simulink model "Automatic_Power_Factor_Correction"  (R2021a)
settings: Solver=ode23tb  StartTime=0.0  StopTime=0.2  RelTol=1e-3
undefined symbols (not defined in the file): D1, Delta
libraries: spsThreePhaseParallelRLCLoadLib x4, spsThreePhaseBreakerLib x3, spsThreePhaseTransformerTwoWindingsLib x1, spsThreePhaseSourceLib x1, spsPower3phInstantaneousLib x1, spsThreePhaseVIMeasurementLib x1, spspowerguiLib x1
settings Model: Creator=thosiba  LastModifiedBy=saman
settings SolverCC: AlgebraicLoopSolver=TrustRegion
settings DataIOCC: ReturnWorkspaceOutputs=off
settings OptimizationCC: LifeSpan=inf
settings DebuggingCC: SFMachineParentedDataDiag=warning  ArithmeticOperatorsInVariantConditions=warning
settings HardwareCC: ProdBitPerSizeT=32  ProdBitPerPtrDiffT=32  ProdWordSize=32  ProdHWDeviceType=Specified
settings SFSimCC: SimUseLocalCustomCode=off  CustomCodeUndefinedFunction=UseInterfaceOnly
settings RTWCC: RTWUseLocalCustomCode=off
settings CodeAppCC: StateflowObjectComments=on
settings SimscapeCC: SimscapeNormalizeSystem=off

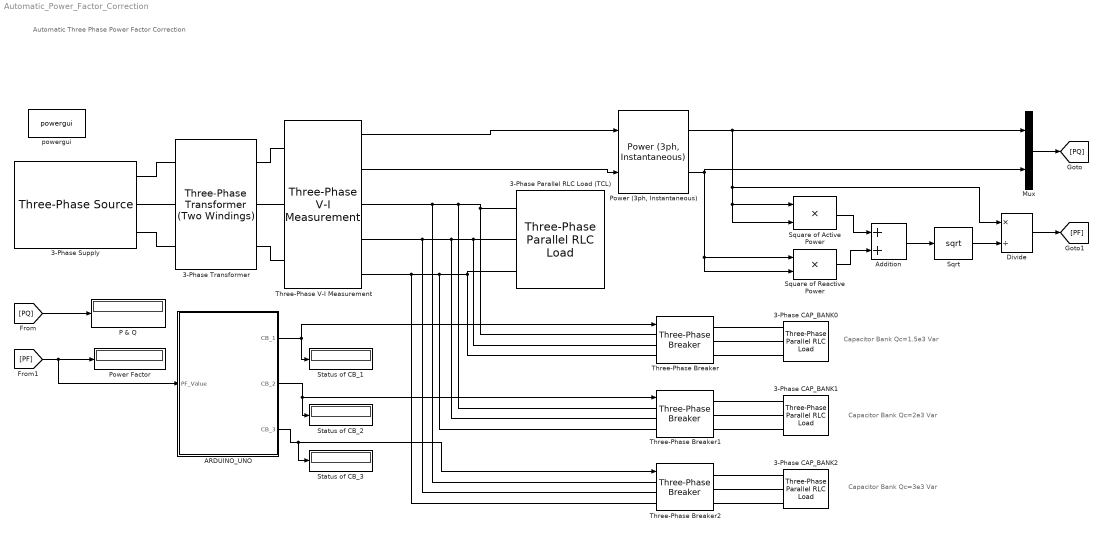
== system Automatic_Power_Factor_Correction ==
  note: Automatic Three Phase Power Factor Correction
  note: Capacitor Bank Qc=1.5e3 Var
  note: Capacitor Bank Qc=2e3 Var
  note: Capacitor Bank Qc=3e3 Var
  3-Phase CAP_BANK0 : spsThreePhaseParallelRLCLoadLib/Three-Phase Parallel RLC Load  LConnTagsString=A|B|C  Configuration=Y (grounded)  NominalVoltage=400  Vabc=[1e3 1e3 1e3]  Vabcp=[1e3 1e3 1e3]  NominalFrequency=50  UnbalancedPower=off  ActivePower=0  InductivePower=0  CapacitivePower=1.5e3  Pabc=[10e3 9e3 11e3]  QLabc=[100 90 110]  QCabc=[100 90 110]  Pabcp=[10e3 9e3 11e3]  QLabcp=[100 90 110]  QCabcp=[100 90 110]  Measurements=None  LoadType=constant PQ
  3-Phase CAP_BANK1 : spsThreePhaseParallelRLCLoadLib/Three-Phase Parallel RLC Load  LConnTagsString=A|B|C  Configuration=Y (grounded)  NominalVoltage=400  Vabc=[1e3 1e3 1e3]  Vabcp=[1e3 1e3 1e3]  NominalFrequency=50  UnbalancedPower=off  ActivePower=0  InductivePower=0  CapacitivePower=2e3  Pabc=[10e3 9e3 11e3]  QLabc=[100 90 110]  QCabc=[100 90 110]  Pabcp=[10e3 9e3 11e3]  QLabcp=[100 90 110]  QCabcp=[100 90 110]  Measurements=None  LoadType=constant PQ
  3-Phase CAP_BANK2 : spsThreePhaseParallelRLCLoadLib/Three-Phase Parallel RLC Load  LConnTagsString=A|B|C  Configuration=Y (grounded)  NominalVoltage=400  Vabc=[1e3 1e3 1e3]  Vabcp=[1e3 1e3 1e3]  NominalFrequency=50  UnbalancedPower=off  ActivePower=0  InductivePower=0  CapacitivePower=3e3  Pabc=[10e3 9e3 11e3]  QLabc=[100 90 110]  QCabc=[100 90 110]  Pabcp=[10e3 9e3 11e3]  QLabcp=[100 90 110]  QCabcp=[100 90 110]  Measurements=None  LoadType=constant PQ
  3-Phase Parallel RLC Load (TCL) : spsThreePhaseParallelRLCLoadLib/Three-Phase Parallel RLC Load  LConnTagsString=A|B|C  Configuration=Y (grounded)  NominalVoltage=400  Vabc=[1e3 1e3 1e3]  Vabcp=[1e3 1e3 1e3]  NominalFrequency=50  UnbalancedPower=off  ActivePower=5e3  InductivePower=7e3  CapacitivePower=0  Pabc=[10e3 9e3 11e3]  QLabc=[100 90 110]  QCabc=[100 90 110]  Pabcp=[10e3 9e3 11e3]  QLabcp=[100 90 110]  QCabcp=[100 90 110]  Measurements=None  LoadType=constant PQ
  "3-Phase Transformer " : spsThreePhaseTransformerTwoWindingsLib/Three-Phase Transformer (Two Windings)  Winding1Connection=Delta (D1)  Winding2Connection=Yg  CoreType=Three single-phase transformers  SetSaturation=off  Hysteresis=off  DataFile='hysteresis'  SetInitialFlux=off  Measurements=None  UNITS=pu  NominalPower=[ 1e6 , 50 ]  Winding1=[ 11e3 , 0.002 , 0.08 ]  Winding2=[ 400 , 0.002 , 0.08 ]  Rm=500  Lm=500  L0=0.5  Saturation=[ 0,0 ; 0.0024,1.2 ; 1.0,1.52 ]  InitialFluxes=[ 0.8 , -0.8 , 0.7 ]  BreakLoop=off  DiscreteSolver=Trapezoidal iterative  DataType=off  TransfoNumber=1
  3-Phase Supply : spsThreePhaseSourceLib/Three-Phase Source  InternalConnection=Yg  VoltagePhases=off  Voltage=11e3  PhaseAngle=0  Voltage_phases=[25e3 25e3 25e3]/sqrt(3)  PhaseAngles_phases=[0 -120 +120]  Frequency=50  NonIdealSource=on  SpecifyImpedance=on  Resistance=0.8929  Inductance=16.58e-3  ShortCircuitLevel=30e6  BaseVoltage=11e3  XRratio=7  BusType=swing  Pref=10e3  Qref=0  Prefabc=[10e3, 10e3, 10e3]  Qrefabc=[0, 0, 0]  Qmin=-inf  Qmax=inf
  ARDUINO_UNO : MATLAB Function  TreatAsAtomicUnit=on
  Addition : Sum
  Divide : Product  Inputs=*/
  Mux : Mux  Inputs=2
  P & Q : Display
      settings: Decimation=4
  "Power (3ph, Instantaneous)" : spsPower3phInstantaneousLib/Power (3ph, Instantaneous)
  Power Factor : Display
      settings: Decimation=4
  Sqrt : Sqrt  SaturateOnIntegerOverflow=on
  Square of Active Power : Product
  Square of Reactive Power : Product
  Status of CB_1 : Display
  Status of CB_2 : Display
  Status of CB_3 : Display
  Three-Phase V-I Measurement : spsThreePhaseVIMeasurementLib/Three-Phase V-I Measurement  VoltageMeasurement=phase-to-ground  SetLabelV=off  LabelV=Vabc  Vpu=off  VpuLL=off  CurrentMeasurement=yes  SetLabelI=off  LabelI=Iabc  Ipu=off  Pbase=100e6  Vbase=500e3  OutputType=Complex  PhasorSimulation=off  PSBequivalent=0
  Three-Phase Breaker : spsThreePhaseBreakerLib/Three-Phase Breaker  InitialState=open  SwitchA=on  SwitchB=on  SwitchC=on  SwitchTimes="[1/60  5/60]"  External=on  BreakerResistance=0.01  SnubberResistance=1e6  SnubberCapacitance=inf  Measurements=None
  Three-Phase Breaker1 : spsThreePhaseBreakerLib/Three-Phase Breaker  InitialState=open  SwitchA=on  SwitchB=on  SwitchC=on  SwitchTimes="[1/60  5/60]"  External=on  BreakerResistance=0.01  SnubberResistance=1e6  SnubberCapacitance=inf  Measurements=None
  Three-Phase Breaker2 : spsThreePhaseBreakerLib/Three-Phase Breaker  InitialState=open  SwitchA=on  SwitchB=on  SwitchC=on  SwitchTimes="[1/60  5/60]"  External=on  BreakerResistance=0.01  SnubberResistance=1e6  SnubberCapacitance=inf  Measurements=None
  powergui : spspowerguiLib/powergui  Priority=1  SimulationMode=Continuous  SampleTime=50e-6  frequency=60  Iterations=50  frequencyindice=50  Pbase=100e6  ErrMax=1e-4  UnitsV=kV  UnitsW=MW  buscounter=0  FunctionMessages=off  echomessages=off  EnableUseOfTLC=off  CurrentSourceSwitches=off  DisableSnubberDevices=off  DisableRonSwitches=off  DisableVfSwitches=off  DisplayEquations=off  AutomaticDiscreteSolvers=off  SolverType=Tustin/Backward Euler (TBE)  Interpol=off  ExternalGateDelay=off  methode=off  Ts=100  x0status=blocks  SPID=off  SwTol=0  HookPort=off  NonlinearTolerance=1e-4  nMaxIteration=100  ContinueOnMaxIteration=off  RestoreLinks=warning  ResistiveCurrentMeasurement=off  Frange=[0:2:500]  Ylog=off  Xlog=on  ShowGrid=off  save=off  variable=ZData  structure=Vpi  ZoomFFT=off  StartTime=0.1  cycles=10  DisplayStyle=1  fundamental=50  FreqAxis=off  MaxFrequency=2000  frequencyindicesteady=1  RmsSteady=1  display=off
  wires:
  Square of Active Power/1 -> Addition/1
  Square of Reactive Power/1 -> Addition/2
  Addition/1 -> Sqrt/1
  Divide/1 -> [PF]
  Sqrt/1 -> Divide/2
  "Power (3ph, Instantaneous)"/1 -> Divide/1, Square of Active Power/2, Square of Active Power/1, Mux/1
  "Power (3ph, Instantaneous)"/2 -> Square of Reactive Power/2, Square of Reactive Power/1, Mux/2
  Mux/1 -> [PQ]
  Three-Phase V-I Measurement/1 -> "Power (3ph, Instantaneous)"/1
  Three-Phase V-I Measurement/2 -> "Power (3ph, Instantaneous)"/2
  [PQ] -> P & Q/1
  [PF] -> Power Factor/1, ARDUINO_UNO/1(PF_Value)
  ARDUINO_UNO/2(CB_2) -> Status of CB_2/1, Three-Phase Breaker1/1
  ARDUINO_UNO/1(CB_1) -> Status of CB_1/1, Three-Phase Breaker/1
  ARDUINO_UNO/3(CB_3) -> Three-Phase Breaker2/1, Status of CB_3/1
  connections:
  "3-Phase Transformer "/RConn1 -- Three-Phase V-I Measurement/LConn1
  "3-Phase Transformer "/RConn2 -- Three-Phase V-I Measurement/LConn2
  "3-Phase Transformer "/RConn3 -- Three-Phase V-I Measurement/LConn3
  3-Phase Supply/RConn3 -- "3-Phase Transformer "/LConn3
  3-Phase Supply/RConn1 -- "3-Phase Transformer "/LConn1
  3-Phase Supply/RConn2 -- "3-Phase Transformer "/LConn2
  3-Phase Parallel RLC Load (TCL)/LConn1 -- Three-Phase Breaker1/LConn1 -- Three-Phase Breaker2/LConn1 -- Three-Phase V-I Measurement/RConn1 -- Three-Phase Breaker/LConn1
  Three-Phase V-I Measurement/RConn2 -- Three-Phase Breaker2/LConn2 -- Three-Phase Breaker1/LConn2 -- Three-Phase Breaker/LConn2 -- 3-Phase Parallel RLC Load (TCL)/LConn2
  Three-Phase V-I Measurement/RConn3 -- Three-Phase Breaker2/LConn3 -- Three-Phase Breaker1/LConn3 -- 3-Phase Parallel RLC Load (TCL)/LConn3 -- Three-Phase Breaker/LConn3
  Three-Phase Breaker/RConn2 -- 3-Phase CAP_BANK0/LConn2
  3-Phase CAP_BANK0/LConn1 -- Three-Phase Breaker/RConn1
  3-Phase CAP_BANK0/LConn3 -- Three-Phase Breaker/RConn3
  3-Phase CAP_BANK1/LConn2 -- Three-Phase Breaker1/RConn2
  3-Phase CAP_BANK1/LConn1 -- Three-Phase Breaker1/RConn1
  3-Phase CAP_BANK1/LConn3 -- Three-Phase Breaker1/RConn3
  3-Phase CAP_BANK2/LConn1 -- Three-Phase Breaker2/RConn1
  Three-Phase Breaker2/RConn2 -- 3-Phase CAP_BANK2/LConn2
  3-Phase CAP_BANK2/LConn3 -- Three-Phase Breaker2/RConn3

== matlab function Automatic_Power_Factor_Correction/ARDUINO_UNO ==
  data: PF_Value input; CB_1 output; CB_2 output; CB_3 output
function [CB_1,CB_2,CB_3] = ARDUINO_UNO(PF_Value)
% Samandar Khan Afridi (19-Electrical)
% Email: samandarkhanafridi@gmail.com
% YouTube: https://www.youtube.com/@samandarkhanafridi

    if (PF_Value<=0.60)
        CB_1=1;
        CB_2=0;
        CB_3=0;
    elseif (PF_Value<=0.75)
        CB_1=0;
        CB_2=1;
        CB_3=0;
    elseif (PF_Value<=0.85)
        CB_1=0;
        CB_2=0;
        CB_3=1;
    else
        CB_1=0;
        CB_2=0;
        CB_3=1;
    end
